simulink model "TestTrigger21a"  (R2021a)
settings: Solver=VariableStepAuto  StartTime=0.0  StopTime=300  RelTol=1e-3
settings Model: EnablePacing=on  Creator=zckog  LastModifiedBy=zckog
settings DebuggingCC: UnconnectedInputMsg=none  UnconnectedOutputMsg=none  UnconnectedLineMsg=none
settings RTWCC: DLArmComputeVersion=20.02.1

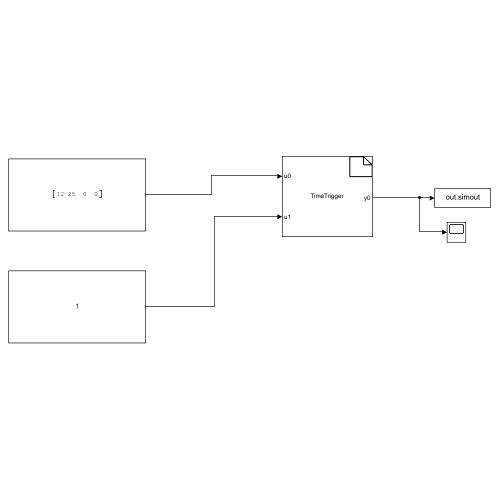
[thumbnail: Simulink's stored preview of the top-level diagram]
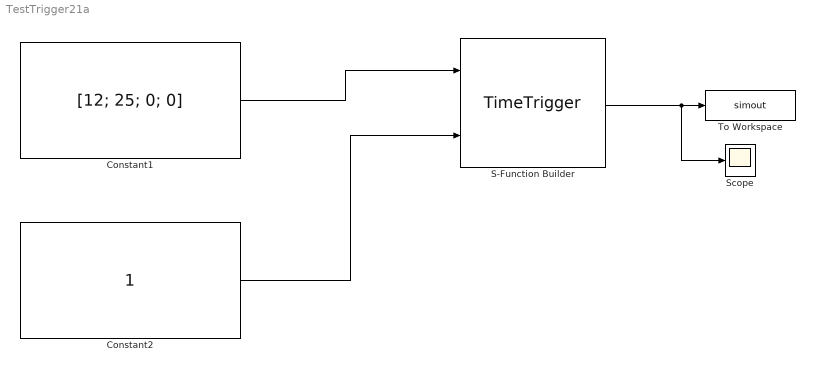
== system TestTrigger21a ==
  Constant1 : Constant  Value=[12; 25; 0; 0]  OutDataTypeStr=int32  SampleTime=1
  Constant2 : Constant  OutDataTypeStr=int32  SampleTime=1
  S-Function Builder : S-Function  FunctionName=TimeTrigger  SFunctionModules=TimeTrigger_wrapper  SFunctionDeploymentMode=off  EnableBusSupport=off  mask(S-Function Builder){}
      mask help: Simulink:masks:SFunctionBuilder_MD
      mask init:
      | val = [[.9  0.75 0.75 1 1 .9 .9 1]',[1 1 0.75 0.75 .9 .9 1 .9]'];try , sys = get_param(gcb,'SfunBuilderFcnName');if isempty(sys), sys = get_param(gcb,'FunctionName'); end,catch, sys = get_param(gcb,'FunctionName'); end
      settings: CopyFcn=set_param(gcbh,'LinkStatus','none')  OpenFcn=sfunctionwizard(gcbh)
      mask Display:
      | plot(val(:,1),val(:,2))
      | disp(sys)
      | port_label('input',1,'u0')
      | port_label('input',2,'u1')
      | port_label('output',1,'y0')
  Scope : Scope
  To Workspace : ToWorkspace  VariableName=simout  SaveFormat=Timeseries  SampleTime=-1
  wires:
  Constant1/1 -> S-Function Builder/1
  Constant2/1 -> S-Function Builder/2
  S-Function Builder/1 -> Scope/1, To Workspace/1
